simulink model "Demo1"  (R2024b)
settings: Solver=VariableStepAuto  StartTime=0.0  StopTime=10  RelTol=1e-3
settings Model: Creator=changeo  LastModifiedBy=misaka10039

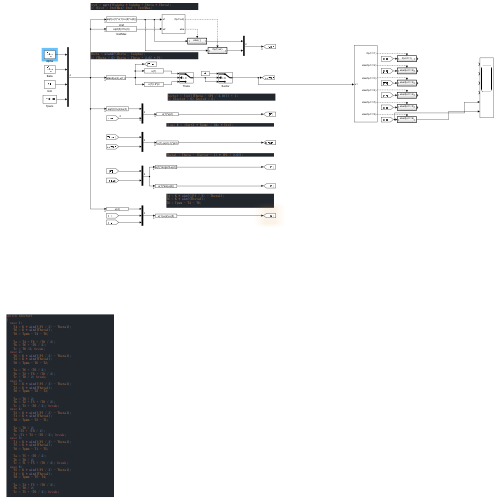
[thumbnail: Simulink's stored preview of the top-level diagram]
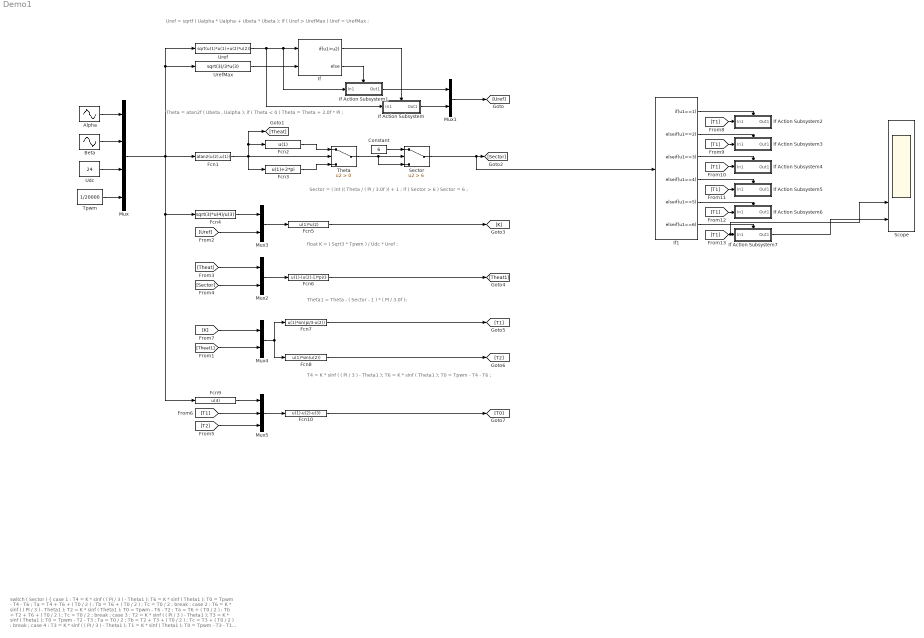
== system Demo1 ==
  note: switch ( Sector )
      | {
      | case 1 :
      | T4 = K * sinf ( ( PI / 3 ) - Theta1 );
      | T6 = K * sinf ( Theta1 );
      | T0 = Tpwm - T4 - T6 ;
      |
      | Ta = T4 + T6 + ( T0 / 2 ) ;
      | Tb = T6 + ( T0 / 2 ) ;
      | Tc = T0 / 2 ; break ;
      | case 2 :
      | T6 = K * sinf ( ( PI / 3 ) - Theta1 );
      | T2 = K * sinf ( Theta1 );
      | T0 = Tpwm - T6 - T2 ;
      |
      | Ta = T6 + ( T0 / 2 ) ;
      | Tb = T2 + T6 + ( T0 / 2 ) ;
      | Tc = T0 / 2 ; break ;
      | case 3 :
      | T2 = K * sinf ( ( PI / 3 ) - Theta1 );
      | T3 = K * sinf ( Theta1 );
      | T0 = Tpwm - T2 - T3 ;
      |
      | Ta = T0 / 2 ;
      | Tb = T2 + T3 + ( T0 / 2 ) ;
      | Tc = T3 + ( T0 / 2 ) ; break ;
      | case 4 :
      | T3 = K * sinf ( ( PI / 3 ) - Theta1 );
      | T1 = K * sinf ( Theta1 );
      | T0 = Tpwm - T3 - T1 ;
      |
      | Ta = T0 / 2 ;
      | Tb = T3 + ( T0 / 2 ) ;
      | Tc = T1 + T3 + ( T0 / 2 ) ; break ;
      | case 5 :
      | T1 = K * sinf ( ( PI / 3 ) - Theta1 );
      | T5 = K * sinf ( Theta1 );
      | T0 = Tpwm - T1 - T5 ;
      |
      | Ta = T5 + ( T0 / 2 ) ;
      | Tb = T0 / 2 ;
      | Tc = T1 + T5 + ( T0 / 2 ) ; break ;
      | case 6 :
      | T5 = K * sinf ( ( PI / 3 ) - Theta1 );
      | T4 = K * sinf ( Theta1 );
      | T0 = Tpwm - T5 - T4 ;
      |
      | Ta = T4 + T5 + ( T0 / 2 ) ;
      | Tb = T0 / 2 ;
      | Tc = T5 + ( T0 / 2 ) ; break ;
      | }
  note: float K = ( Sqrt3 * Tpwm ) / Udc * Uref ;
  note: Theta1 = Theta - ( Sector - 1 ) * ( PI / 3.0f );
  note: Sector = ( int )( Theta / ( PI / 3.0f )) + 1 ;
      | if ( Sector > 6 ) Sector = 6 ;
  note: Theta = atan2f ( Ubeta , Ualpha );
      | if ( Theta < 0 ) Theta = Theta + 2.0f * PI ;
  note: Uref = sqrtf ( Ualpha * Ualpha + Ubeta * Ubeta );
      | if ( Uref > UrefMax ) Uref = UrefMax ;
  note: T4 = K * sinf ( ( PI / 3 ) - Theta1 );
      | T6 = K * sinf ( Theta1 );
      | T0 = Tpwm - T4 - T6 ;
  Alpha : Sin  Amplitude=5  Frequency=100  SampleTime=0
  Beta : Sin  Amplitude=10  Frequency=100  Phase=pi/2  SampleTime=0
  Constant : Constant  Value=6
  Fcn1 : Fcn  Expr=atan2(u(2),u(1))
  Fcn10 : Fcn  Expr=u(1)-u(2)-u(3)
  Fcn2 : Fcn  Expr=u(1)
  Fcn3 : Fcn  Expr=u(1)+2*pi
  Fcn4 : Fcn  Expr=sqrt(3)*u(4)/u(3)
  Fcn5 : Fcn  Expr=u(1)*u(2)
  Fcn6 : Fcn  Expr=u(1)-(u(2)-1)*pi/3
  Fcn7 : Fcn  Expr=u(1)*sin(pi/3-u(2))
  Fcn8 : Fcn  Expr=u(1)*sin(u(2))
  Fcn9 : Fcn  Expr=u(4)
  If : If  NumInputs=2  IfExpression=u1>u2
  If Action Subsystem : Subsystem  TreatAsAtomicUnit=on
  If Action Subsystem1 : Subsystem  TreatAsAtomicUnit=on
  If Action Subsystem2 : Subsystem  TreatAsAtomicUnit=on
  If Action Subsystem3 : Subsystem  TreatAsAtomicUnit=on
  If Action Subsystem4 : Subsystem  TreatAsAtomicUnit=on
  If Action Subsystem5 : Subsystem  TreatAsAtomicUnit=on
  If Action Subsystem6 : Subsystem  TreatAsAtomicUnit=on
  If Action Subsystem7 : Subsystem  TreatAsAtomicUnit=on
  If1 : If  IfExpression=u1==1  ElseIfExpressions=u1==2,u1==3,u1==4,u1==5,u1==6  ShowElse=off
  Mux : Mux
  Mux{1..4} (4 alike) : Mux  Inputs=2
  Mux5 : Mux  Inputs=3
  Scope : Scope  NumInputPorts=6
  Sector : Switch  Criteria=u2 > Threshold  Threshold=6  SaturateOnIntegerOverflow=off  InputSameDT=off
  Theta : Switch  Criteria=u2 > Threshold  SaturateOnIntegerOverflow=off  InputSameDT=off
  Tpwm : Constant  Value=1/20000
  Udc : Constant  Value=24
  Uref : Fcn  Expr=sqrt(u(1)*u(1)+u(2)*u(2))
  UrefMax : Fcn  Expr=sqrt(3)/3*u(3)
  wires:
  Alpha/1 -> Mux/1
  Beta/1 -> Mux/2
  Udc/1 -> Mux/3
  Tpwm/1 -> Mux/4
  Mux/1 -> Fcn9/1, Fcn4/1, UrefMax/1, Uref/1, Fcn1/1
  UrefMax/1 -> If/2
  If/1 -> If Action Subsystem/Action
  If/2 -> If Action Subsystem1/Action
  If Action Subsystem1/1(Out1) -> Mux1/1
  If Action Subsystem/1(Out1) -> Mux1/2
  Mux1/1 -> [Uref]
  Constant/1 -> Sector/1
  Fcn3/1 -> Theta/3
  Theta/1 -> Sector/3, Sector/2
  Fcn2/1 -> Theta/1
  Fcn1/1 -> Fcn2/1, [Theat], Fcn3/1, Theta/2
  Fcn4/1 -> Mux3/1
  [Uref] -> Mux3/2
  [Sector] -> Mux2/2
  Mux3/1 -> Fcn5/1
  Fcn5/1 -> [K]
  Mux2/1 -> Fcn6/1
  [Theat] -> Mux2/1
  [T2] -> Mux5/3
  Mux5/1 -> Fcn10/1
  Fcn6/1 -> [Theat1]
  [K] -> Mux4/1
  [Theat1] -> Mux4/2
  Mux4/1 -> Fcn8/1, Fcn7/1
  Fcn9/1 -> Mux5/1
  Fcn8/1 -> [T2]
  Uref/1 -> If Action Subsystem/1(In1), If Action Subsystem1/1(In1), If/1
  Fcn10/1 -> [T0]
  [T1] -> Mux5/2
  Fcn7/1 -> [T1]
  Sector/1 -> If1/1, [Sector]
  If1/1 -> If Action Subsystem2/Action
  [T1] -> If Action Subsystem2/1(In1)
  [T1] -> If Action Subsystem3/1(In1)
  If1/2 -> If Action Subsystem3/Action
  If1/3 -> If Action Subsystem4/Action
  [T1] -> If Action Subsystem4/1(In1)
  [T1] -> If Action Subsystem5/1(In1)
  If1/4 -> If Action Subsystem5/Action
  If1/5 -> If Action Subsystem6/Action
  [T1] -> If Action Subsystem6/1(In1)
  [T1] -> Scope/5, If Action Subsystem7/1(In1)
  If1/6 -> If Action Subsystem7/Action
  If Action Subsystem7/1(Out1) -> Scope/6

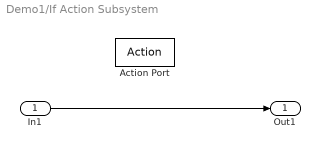
== system Demo1/If Action Subsystem ==
  In1 : Inport
  Action Port : ActionPort  ActionPortLabel=if(u1>u2)
  Out1 : Outport
  wires:
  In1/1 -> Out1/1

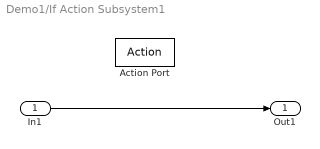
== system Demo1/If Action Subsystem1 ==
  In1 : Inport
  Action Port : ActionPort  ActionPortLabel=else
  Out1 : Outport
  wires:
  In1/1 -> Out1/1

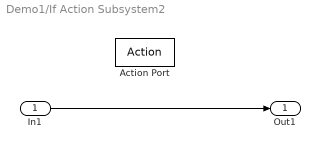
== system Demo1/If Action Subsystem2 ==
  In1 : Inport
  Action Port : ActionPort  ActionPortLabel=if(u1==1)
  Out1 : Outport
  wires:
  In1/1 -> Out1/1

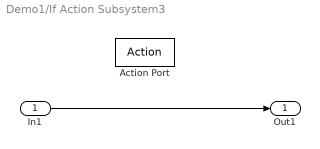
== system Demo1/If Action Subsystem3 ==
  In1 : Inport
  Action Port : ActionPort  ActionPortLabel=elseif(u1==2)
  Out1 : Outport
  wires:
  In1/1 -> Out1/1

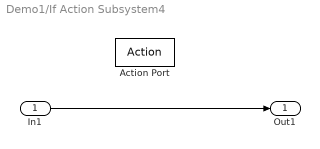
== system Demo1/If Action Subsystem4 ==
  In1 : Inport
  Action Port : ActionPort  ActionPortLabel=elseif(u1==3)
  Out1 : Outport
  wires:
  In1/1 -> Out1/1

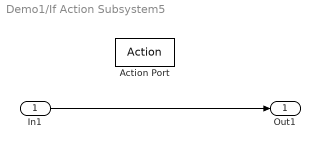
== system Demo1/If Action Subsystem5 ==
  In1 : Inport
  Action Port : ActionPort  ActionPortLabel=elseif(u1==4)
  Out1 : Outport
  wires:
  In1/1 -> Out1/1

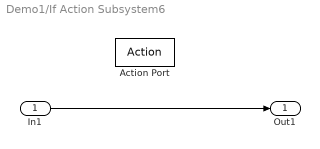
== system Demo1/If Action Subsystem6 ==
  In1 : Inport
  Action Port : ActionPort  ActionPortLabel=elseif(u1==5)
  Out1 : Outport
  wires:
  In1/1 -> Out1/1

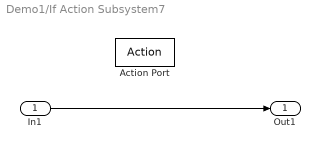
== system Demo1/If Action Subsystem7 ==
  In1 : Inport
  Action Port : ActionPort  ActionPortLabel=elseif(u1==6)
  Out1 : Outport
  wires:
  In1/1 -> Out1/1
